simulink model "sysgenDDC"  (Simulink 7.7)
settings: Solver=VariableStepDiscrete  SolverMode=SingleTasking  StartTime=0.0  StopTime=0.003  RelTol=1e-3
PreLoadFcn:
  | sysgenDDC_PreLoadFcn
values from neighbouring files (symbols this model uses):
  Gz = [  340 ... (first row only)    [sysgenDDC_PreLoadFcn.m]
  Hz = [479 ... (first row only)    [sysgenDDC_PreLoadFcn.m]
  Ts = 1/40e006    (= 2.5e-08)    [sysgenDDC_PreLoadFcn.m]
undefined symbols (not defined in the file or in its folder): get, One, sided, xlGetSimulinkPeriod, xlipgetpartsetting
libraries: xbsIndex_r4 x132, dspsnks4 x2, xbsCopyrightNotice_r4 x1
(part 1 of 2)
settings Model: Creator=alexc  LastModifiedBy=douangp
settings DataIOCC: SignalLoggingName=sigsOut
settings OptimizationCC: BlockReduction=off  BooleanDataType=off  InitFltsAndDblsToZero=on
settings DebuggingCC: SaveWithParameterizedLinksMsg=none  SignalResolutionControl=TryResolveAllWithWarning  SolverPrmCheckMsg=none  MultiTaskDSMMsg=warning  MultiTaskCondExecSysMsg=none  StrictBusMsg=None
settings HardwareCC: TargetUnknown=on
settings RTWCC: IncludeERTFirstTime=on
settings GRTTargetCC: TargetFcnLib=ansi_tfl_tmw.mat

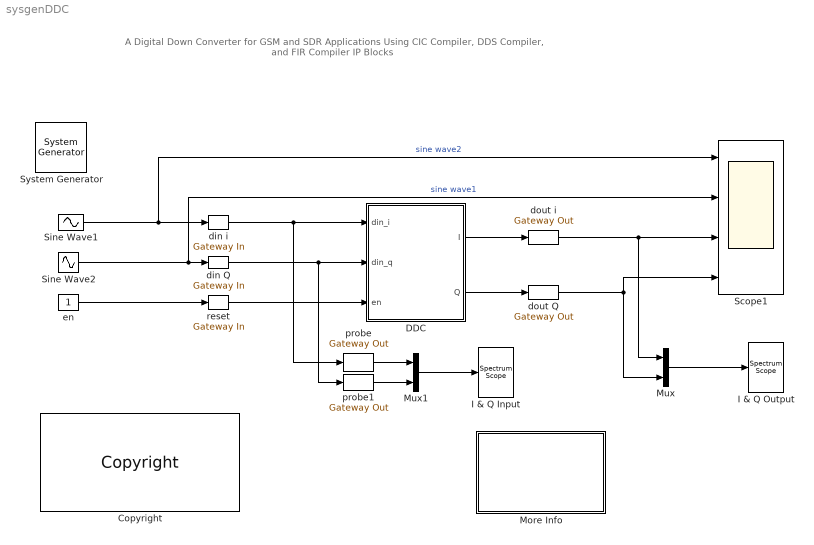
== system sysgenDDC ==
  note: A Digital Down Converter for GSM and SDR Applications
      | Using CIC Compiler, DDS Compiler, and FIR Compiler IP Blocks
  " System Generator" : xbsIndex_r4/ System Generator  Tag=genX  SystemSampleTime=-1  xilinxfamily=virtex6  part=xc6vlx240t  speed=-1  package=ff1156  synthesis_tool=XST  clock_wrapper=Clock Enables  directory=./netlist  proj_type=Project Navigator  Synth_file=XST Defaults  Impl_file=ISE Defaults  testbench=off  simulink_period=Ts  sysclk_period=6  dcm_input_clock_period=100  incr_netlist=off  trim_vbits=Everywhere in SubSystem  dbl_ovrd=According to Block Masks  core_generation=According to Block Masks  run_coregen=off  deprecated_control=off  eval_field=0  block_type=sysgen
      settings: block_version=10.1.3
  Copyright : xbsCopyrightNotice_r4/Copyright  copyrighttext="Copyright (c) 2011  by  Xilinx, Inc. All rights reserved.<br><br>This file contains proprietary, confidential information of Xilinx, Inc., is distributed under license from Xilinx, Inc., and may be used, copied and/or disclosed only pursuant to the terms of a valid license agreement with Xilinx, Inc. Xilinx hereby grants you a license to use this file solely for design, simulation, implementation and creation of design files limited to Xilinx devices or technologies. Use with non-Xilinx devices or technologies is expressly prohibited and immediately terminates your license unless covered by a separate agreement.<br><br>Xilinx is providing this design, code, or information \"as-is\" solely for use in developing programs and solutions for Xilinx devices, with no obligation on the part of Xilinx to provide support. By providing this design, code, or information as one possible implementation of this feature, application or standard, Xilinx is making no representation that this implementation is free from any claims of infringement. You are responsible for obtaining any rights you may require for your implementation. Xilinx expressly disclaims any warranty whatsoever with respect to the adequacy of the implementation, including but not limited to any warranties or representations that this implementation is free from claims of infringement, implied warranties of merchantability or fitness for a particular purpose.<br><br>Xilinx products are not intended for use in life support appliances, devices, or systems. Use in such applications is expressly prohibited.<br><br>Any modifications that are made to the Source Code are done at the user's sole risk and will be unsupported.<br><br>This copyright and support notice must be retained as part of this text at all times. (c) Copyright 1995-2011 Xilinx, Inc. All rights reserved."  block_type=copyright
      settings: block_version=9.2.00
      settings: infoedit=|
      | Copyright(C) 2007 by  Xilinx, Inc. All rights reserved.<br>
      | <br>
      | This file contains proprietary, confidential information of Xilinx, Inc., is distributed under license
      | from Xilinx, Inc., and may be used, copied and/or disclosed only pursuant to the terms of a valid license
      | agreement with Xilinx, Inc. Xilinx hereby grants you a license to use this file solely for design,
      | simulation, implementation and creation of design files limited to Xilinx devices or technologies. Use
      | with non-Xilinx devices or technologies is expressly prohibited and immediately terminates your license
      | unless covered by a separate agreement.<br>
      | <br>
      | Xilinx is providing this design, code, or information "as-is" solely for use in developing programs and
      | solutions for Xilinx devices, with no obligation on the part of Xilinx to provide support. By providing
      | this design, code, or information as one possible implementation of this feature, application or standard,
      | Xilinx is making no representation that this implementation is free from any claims of infringement. You
      | are responsible for obtaining any rights you may require for your implementation. Xilinx expressly disclaims
      | any warranty whatsoever with respect to the adequacy of the implementation, including but not limited to any
      | warranties or representations that this implementation is free from claims of infringement, implied warranties
      | of merchantability or fitness for a particular purpose.<br>
      | <br>
      | Xilinx products are not intended for use in life support appliances, devices, or systems. Use in such
      | applications is expressly prohibited.<br>
      | <br>
      | Any modifications that are made to the Source Code are done at the user's sole risk and will be unsupported.<br>
      | <br>
      | This copyright and support notice must be retained as part of this text at all times.
      | (c) Copyright 1995-2007 Xilinx, Inc. All rights reserved.
  DDC : Subsystem
  I & Q Input : dspsnks4/Spectrum Scope  SystemSampleTime=-1  ScopeProperties=off  Domain=Frequency  HorizSpan=1  UseBuffer=on  BufferSize=512  Overlap=64  TreatMby1Signals=M channels  inpFftLenInherit=off  FFTlength=128  numAvg=2  DisplayProperties=off  AxisGrid=on  Memory=off  FrameNumber=on  AxisLegend=on  AxisZoom=off  OpenScopeAtSimStart=on  OpenScopeImmediately=off  FigPos=get(0,'defaultfigureposition')  AxisProperties=on  XUnits=Hertz  XRange=One-sided ([0...Fs/2])  XDisplay=0  InheritXIncr=off  XIncr=1.0  XLabel=Samples  XLimit=Auto  YUnits=dBW/Hertz  XMax=1  XMin=0  YLabel=Magnitude, dB  LineProperties=off  LineMarkers=+  LineColors=[0 0 1]|[1 0 0]  wintypeSpecScope=Hann  RsSpecScope=50  betaSpecScope=5  winsampSpecScope=Periodic  XAxisParamsVer=6.8  isFrameUpgraded=on
      settings: YMin=-103.063615575883  YMax=27.7949833359379
  I & Q Output : dspsnks4/Spectrum Scope  SystemSampleTime=-1  ScopeProperties=off  Domain=Frequency  HorizSpan=1  UseBuffer=on  BufferSize=512  Overlap=64  TreatMby1Signals=M channels  inpFftLenInherit=off  FFTlength=128  numAvg=2  DisplayProperties=off  AxisGrid=on  Memory=off  FrameNumber=on  AxisLegend=off  AxisZoom=off  OpenScopeAtSimStart=on  OpenScopeImmediately=off  FigPos=get(0,'defaultfigureposition')  AxisProperties=on  XUnits=Hertz  XRange=One-sided ([0...Fs/2])  XDisplay=0  InheritXIncr=off  XIncr=1.0  XLabel=Samples  XLimit=Auto  YUnits=dBW/Hertz  XMax=1  XMin=0  YLabel=Magnitude, dB  LineProperties=off  LineDisables=on|on  LineStyles=--  LineMarkers=None|None  LineColors=[0 0 1]|[1 0 0]  wintypeSpecScope=Hann  RsSpecScope=50  betaSpecScope=5  winsampSpecScope=Periodic  XAxisParamsVer=6.8  isFrameUpgraded=on
      settings: YMin=-103.063615575883  YMax=27.7949833359379
  More Info : Subsystem
      mask Display: disp('Double click\n for\n more information.')
  Mux : Mux  Inputs=2
  Mux1 : Mux  Inputs=2
  Scope1 : Scope  NumInputPorts=4
      settings: TickLabels=on  YMin=-5.5e-005~-0.00025~-1~-1  YMax=0~0~1~1  SaveName=ScopeData3
  Sine Wave1 : Sin  Amplitude=1.9  Frequency=2*pi*4.975e06  SampleTime=Ts
  Sine Wave2 : Sin  Amplitude=1.9  Frequency=2*pi*5.015e06  SampleTime=Ts
  din Q : xbsIndex_r4/Gateway In  gui_display_data_type=Fixed-point  arith_type="Signed  (2's comp)"  n_bits=14  bin_pt=12  preci_type=Single  exp_width=8  frac_width=24  quantization="Round  (unbiased: +/- Inf)"  overflow=Flag as error  period=Ts  dbl_ovrd=off  timing_constraint=None  locs_specified=off  LOCs={}  hdl_port=on  block_type=gatewayin
      settings: infoedit="Gateway in block.  Converts inputs of type Simulink integer, double and fixed point to  Xilinx fixed point type.<br><br>Hardware notes:  In hardware these blocks become top level input ports."  xl_area=[0 0 0 0 14 0 0]  block_version=VER_STRING_GOES_HERE
  din i : xbsIndex_r4/Gateway In  gui_display_data_type=Fixed-point  arith_type="Signed  (2's comp)"  n_bits=14  bin_pt=12  preci_type=Single  exp_width=8  frac_width=24  quantization="Round  (unbiased: +/- Inf)"  overflow=Flag as error  period=Ts  dbl_ovrd=off  timing_constraint=None  locs_specified=off  LOCs={}  hdl_port=on  block_type=gatewayin
      settings: infoedit="Gateway in block.  Converts inputs of type Simulink integer, double and fixed point to  Xilinx fixed point type.<br><br>Hardware notes:  In hardware these blocks become top level input ports."  xl_area=[0 0 0 0 14 0 0]  block_version=VER_STRING_GOES_HERE
  dout Q : xbsIndex_r4/Gateway Out  hdl_port=on  timing_constraint="Data Rate;  Set 'FAST' Attribute"  locs_specified=off  LOCs={}  block_type=gatewayout
      settings: infoedit="Gateway out block.  Converts Xilinx fixed point inputs into ouputs of type Simulink integer, double, or fixed point.<P><P>Hardware notes:  In hardware these blocks become top level output ports or are discarded, depending on how they are configured."  xl_area=[0 0 0 0 20 0 0]  block_version=VER_STRING_GOES_HERE
  dout i : xbsIndex_r4/Gateway Out  hdl_port=on  timing_constraint="Data Rate;  Set 'FAST' Attribute"  locs_specified=off  LOCs={}  block_type=gatewayout
      settings: infoedit="Gateway out block.  Converts Xilinx fixed point inputs into ouputs of type Simulink integer, double, or fixed point.<P><P>Hardware notes:  In hardware these blocks become top level output ports or are discarded, depending on how they are configured."  xl_area=[0 0 0 0 20 0 0]  block_version=VER_STRING_GOES_HERE
  en : Constant  SampleTime=Ts
  probe : xbsIndex_r4/Gateway Out  hdl_port=off  timing_constraint="Data Rate;  Set 'FAST' Attribute"  locs_specified=off  LOCs={}  block_type=gatewayout
      settings: infoedit="Gateway out block.  Converts Xilinx fixed point inputs into ouputs of type Simulink integer, double, or fixed point.<P><P>Hardware notes:  In hardware these blocks become top level output ports or are discarded, depending on how they are configured."  xl_area=[0 0 0 0 0 0 0]  block_version=VER_STRING_GOES_HERE
  probe1 : xbsIndex_r4/Gateway Out  hdl_port=off  timing_constraint="Data Rate;  Set 'FAST' Attribute"  locs_specified=off  LOCs={}  block_type=gatewayout
      settings: infoedit="Gateway out block.  Converts Xilinx fixed point inputs into ouputs of type Simulink integer, double, or fixed point.<br><br>Hardware notes:  In hardware these blocks become top level output ports or are discarded, depending on how they are configured."  xl_area=[0 0 0 0 0 0 0]  block_version=VER_STRING_GOES_HERE
  reset : xbsIndex_r4/Gateway In  gui_display_data_type=Fixed-point  arith_type=Boolean  n_bits=24  bin_pt=0  preci_type=Single  exp_width=8  frac_width=24  quantization=Truncate  overflow=Wrap  period=Ts  dbl_ovrd=off  timing_constraint=None  locs_specified=off  LOCs={}  hdl_port=on  block_type=gatewayin
      settings: infoedit="Gateway in block.  Converts inputs of type Simulink integer, double and fixed point to  Xilinx fixed point type.<br><br>Hardware notes:  In hardware these blocks become top level input ports."  block_version=VER_STRING_GOES_HERE
  wires:
  Sine Wave1/1 -> Scope1/1, din i/1  "sine wave2"
  DDC/1(I) -> dout i/1
  DDC/2(Q) -> dout Q/1
  Sine Wave2/1 -> din Q/1, Scope1/2  "sine wave1"
  din Q/1 -> DDC/2(din_q), probe1/1
  din i/1 -> probe/1, DDC/1(din_i)
  dout i/1 -> Scope1/3, Mux/1
  dout Q/1 -> Scope1/4, Mux/2
  Mux/1 -> I & Q Output/1
  Mux1/1 -> I & Q Input/1
  probe/1 -> Mux1/1
  probe1/1 -> Mux1/2
  en/1 -> reset/1
  reset/1 -> DDC/3(en)

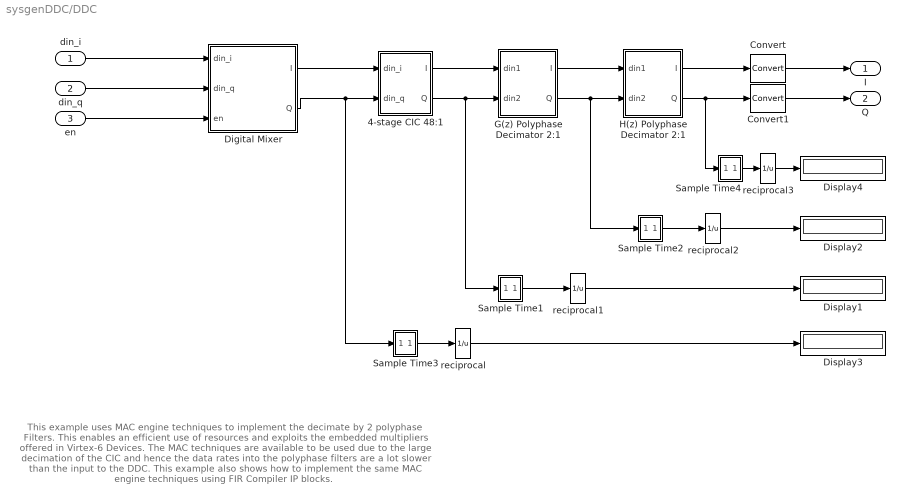
== system sysgenDDC/DDC ==
  note: This example uses MAC engine techniques to implement the decimate by 2
      | polyphase Filters. This enables an efficient use of resources and exploits the
      | embedded multipliers offered in Virtex-6 Devices. The MAC techniques are
      | available to be used due to the large decimation of the CIC and hence the data
      | rates into the polyphase filters are a lot slower than the input to the DDC.
      |
      | This example also shows how to implement the same MAC engine techniques using
      | FIR Compiler IP blocks.
  din_i : Inport
  din_q : Inport  Port=2
  en : Inport  Port=3
  4-stage CIC 48:1 : Subsystem
      mask init:
      | % Set Block Logo
      | bg = [0.3 0.8 0.3];
      | fg = [0.8 1 0.8];
      | iPos = get_param(gcb,'Position');
      | iWidth=iPos(3)-iPos(1); iHeight=iPos(4)-iPos(2);
      | iCx=iWidth/2;
      | iCy=iHeight/2;
      | [logoX, logoY] = xlogo(iPos);
      mask Display:
      | patch([0 iWidth iWidth 0],[0 0 iHeight iHeight] , bg);
      | patch(logoX,logoY , fg);
      | plot([0 0 iWidth iWidth 0], [0 iHeight iHeight 0 0]);
      | 
      | port_label('output',1,'I');
      | port_label('output',2,'Q');
  Convert : xbsIndex_r4/Convert  gui_display_data_type=Fixed-point  arith_type="Signed  (2's comp)"  n_bits=20  bin_pt=18  float_type=Single  exp_bits=8  fraction_bits=24  quantization="Round  (unbiased: +/- Inf)"  overflow=Flag as error  en=off  latency=1  dbl_ovrd=off  pipeline=off  block_type=convert
      settings: xl_area=[11 20 0 22 0 0 0]  block_version=VER_STRING_GOES_HERE
  Convert1 : xbsIndex_r4/Convert  gui_display_data_type=Fixed-point  arith_type="Signed  (2's comp)"  n_bits=20  bin_pt=18  float_type=Single  exp_bits=8  fraction_bits=24  quantization="Round  (unbiased: +/- Inf)"  overflow=Flag as error  en=off  latency=1  dbl_ovrd=off  pipeline=off  block_type=convert
      settings: xl_area=[11 20 0 22 0 0 0]  block_version=VER_STRING_GOES_HERE
  Digital Mixer : Subsystem
      mask init:
      | % Set Block Logo
      | bg = [0.3 0.8 0.3];
      | fg = [0.8 1 0.8];
      | iPos = get_param(gcb,'Position');
      | iWidth=iPos(3)-iPos(1); iHeight=iPos(4)-iPos(2);
      | iCx=iWidth/2;
      | iCy=iHeight/2;
      | [logoX, logoY] = xlogo(iPos);
      mask Display:
      | patch([0 iWidth iWidth 0],[0 0 iHeight iHeight] , bg);
      | patch(logoX,logoY , fg);
      | plot([0 0 iWidth iWidth 0], [0 iHeight iHeight 0 0]);
      | 
      | port_label('input',1,'din');
      | port_label('input',2,'din');
      | port_label('output',1,'I');
      | port_label('output',2,'Q');
  Display{1..4} (4 alike) : Display
  G(z) Polyphase Decimator 2:1 : Subsystem
      mask init:
      | % Set Block Logo
      | bg = [0.3 0.8 0.3];
      | fg = [0.8 1 0.8];
      | iPos = get_param(gcb,'Position');
      | iWidth=iPos(3)-iPos(1); iHeight=iPos(4)-iPos(2);
      | iCx=iWidth/2;
      | iCy=iHeight/2;
      | [logoX, logoY] = xlogo(iPos);
      mask Display:
      | patch([0 iWidth iWidth 0],[0 0 iHeight iHeight] , bg);
      | patch(logoX,logoY , fg);
      | plot([0 0 iWidth iWidth 0], [0 iHeight iHeight 0 0]);
      | 
      | port_label('output',1,'I');
      | port_label('output',2,'Q');
  H(z) Polyphase Decimator 2:1 : Subsystem
      mask init:
      | % Set Block Logo
      | bg = [0.3 0.8 0.3];
      | fg = [0.8 1 0.8];
      | iPos = get_param(gcb,'Position');
      | iWidth=iPos(3)-iPos(1); iHeight=iPos(4)-iPos(2);
      | iCx=iWidth/2;
      | iCy=iHeight/2;
      | [logoX, logoY] = xlogo(iPos);
      mask Display:
      | patch([0 iWidth iWidth 0],[0 0 iHeight iHeight] , bg);
      | patch(logoX,logoY , fg);
      | plot([0 0 iWidth iWidth 0], [0 iHeight iHeight 0 0]);
      | 
      | port_label('output',1,'I');
      | port_label('output',2,'Q');
  Sample Time1 : Subsystem
      settings: CopyFcn=set_param(gcb, 'LinkStatus', 'none');
      mask Display: disp('ST')
  Sample Time2 : Subsystem
      settings: CopyFcn=set_param(gcb, 'LinkStatus', 'none');
      mask Display: disp('ST')
  Sample Time3 : Subsystem
      settings: CopyFcn=set_param(gcb, 'LinkStatus', 'none');
      mask Display: disp('ST')
  Sample Time4 : Subsystem
      settings: CopyFcn=set_param(gcb, 'LinkStatus', 'none');
      mask Display: disp('ST')
  reciprocal{,1..3} (4 alike) : Math  Operator=reciprocal  SaturateOnIntegerOverflow=on
  I : Outport
  Q : Outport  Port=2
  wires:
  Digital Mixer/1(I) -> 4-stage CIC 48:1/1(din_i)
  Digital Mixer/2(Q) -> 4-stage CIC 48:1/2(din_q), Sample Time3/1(din)
  4-stage CIC 48:1/2(Q) -> Sample Time1/1(din), G(z) Polyphase Decimator 2:1/2(din2)
  Sample Time3/1(CLK) -> reciprocal/1
  Sample Time2/1(CLK) -> reciprocal2/1
  din_i/1 -> Digital Mixer/1(din_i)
  din_q/1 -> Digital Mixer/2(din_q)
  Sample Time4/1(CLK) -> reciprocal3/1
  reciprocal/1 -> Display3/1
  H(z) Polyphase Decimator 2:1/2(Q) -> Sample Time4/1(din), Convert1/1
  H(z) Polyphase Decimator 2:1/1(I) -> Convert/1
  Sample Time1/1(CLK) -> reciprocal1/1
  reciprocal1/1 -> Display1/1
  reciprocal2/1 -> Display2/1
  reciprocal3/1 -> Display4/1
  en/1 -> Digital Mixer/3(en)
  G(z) Polyphase Decimator 2:1/2(Q) -> Sample Time2/1(din), H(z) Polyphase Decimator 2:1/2(din2)
  G(z) Polyphase Decimator 2:1/1(I) -> H(z) Polyphase Decimator 2:1/1(din1)
  4-stage CIC 48:1/1(I) -> G(z) Polyphase Decimator 2:1/1(din1)
  Convert1/1 -> Q/1
  Convert/1 -> I/1

== system sysgenDDC/More Info ==
  note: Virtually all digital receivers perform channel access using a digital down-converter (DDC).
      |
      | The desired channel is translated to baseband using the digital mixer comprised
      | of multipliers, M1 and M2, and a direct digital synthesizer (DDS Compiler).  The sample rate of the
      | signal is then adjusted to match the channel bandwidth.  This is performed using a
      | multi-stage multi-rate filter consisting of  CIC Compier Filters and two polyphase decimators.  Coefficients
      | to two poyphase decimator filters are supplied by the MATLAB file (sysgenDDC_PreLoadFcn.m) and preloaded
      | when the model is open.
      |
      | The functions performed in the system are as follows:
      |   -  Waveform synthesis (DDS Compiler)
      |   - Complex multiplication
      |   - Multi-rate filtering with a combination of DDS Compiler and Polyphase decimators.
      |
      | The overall sample rate change of the DDC is 192 (48 x 2 x 2).
      | The DDS mixer signal has a spurious free dynamic range (SFDR) of 96 dB using Phase Dithering correction.
  note: A Digital Down Converter for GSM and SDR Applications

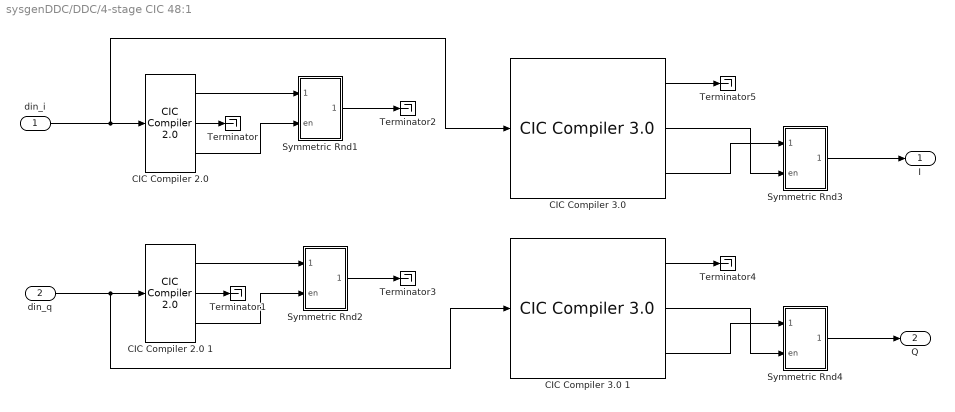
== system sysgenDDC/DDC/4-stage CIC 48:1 ==
  din_i : Inport
  din_q : Inport  Port=2
  "CIC Compiler 2.0 " : xbsIndex_r4/CIC Compiler 2.0   filter_type=Decimation  number_of_stages=4  differential_delay=1  number_of_channels=1  sample_rate_changes=Fixed  fixed_or_initial_rate=48  minimum_rate=48  maximum_rate=48  ratespecification=Maximum_Possible  sampleperiod=1  hardwareoversamplingrate=1  quantization=Full_Precision  output_data_width=41  use_xtreme_dsp_slice=on  use_streaming_interface=on  sclr=off  ce=off  gui_behaviour=Sysgen  input_data_width=18  ip_name=CIC Compiler  ip_version=2.0  dsptool_ready=true  wrapper_available=true  port_translation_map={ 'ce' => 'en', 'sclr' => 'rst' }  ipcore_xco_need_fpga_part=true  ipcore_fpga_part=xlipgetpartsetting(gcb, {'virtex4', 'xc4vsx35', '-10', 'ff668'})  ipcore_verbose=false  block_type=cic_compiler_v2_0
      settings: block_version=12.1
  CIC Compiler 2.0 1 : xbsIndex_r4/CIC Compiler 2.0   filter_type=Decimation  number_of_stages=4  differential_delay=1  number_of_channels=1  sample_rate_changes=Fixed  fixed_or_initial_rate=48  minimum_rate=4  maximum_rate=4  ratespecification=Maximum_Possible  sampleperiod=1  hardwareoversamplingrate=1  quantization=Full_Precision  output_data_width=26  use_xtreme_dsp_slice=on  use_streaming_interface=on  sclr=off  ce=off  gui_behaviour=Sysgen  input_data_width=18  ip_name=CIC Compiler  ip_version=2.0  dsptool_ready=true  wrapper_available=true  port_translation_map={ 'ce' => 'en', 'sclr' => 'rst' }  ipcore_xco_need_fpga_part=true  ipcore_fpga_part=xlipgetpartsetting(gcb, {'virtex4', 'xc4vsx35', '-10', 'ff668'})  ipcore_verbose=false  block_type=cic_compiler_v2_0
      settings: block_version=12.1
  "CIC Compiler 3.0 " : xbsIndex_r4/CIC Compiler 3.0   filter_type=Decimation  number_of_stages=4  differential_delay=1  number_of_channels=1  sample_rate_changes=Fixed  fixed_or_initial_rate=48  minimum_rate=48  maximum_rate=48  ratespecification=Maximum_Possible  sampleperiod=1  hardwareoversamplingrate=1  quantization=Full_Precision  output_data_width=41  use_xtreme_dsp_slice=on  use_streaming_interface=on  has_aclken=off  has_aresetn=off  has_dout_tready=off  trim_axipin_name=on  gui_behaviour=Sysgen_GUI  input_data_width=18  ip_name=CIC Compiler  ip_version=3.0  dsptool_ready=true  wrapper_available=true  port_translation_map={ 'aclken' => 'en', 'aresetn' => 'rst' }  ipcore_xco_need_fpga_part=true  ipcore_fpga_part=xlipgetpartsetting(gcb, {'virtex7', 'xc7v1500t', '-2', 'fhg1157'})  ipcore_verbose=false  block_type=cic_compiler_v3_0
  CIC Compiler 3.0 1 : xbsIndex_r4/CIC Compiler 3.0   filter_type=Decimation  number_of_stages=4  differential_delay=1  number_of_channels=1  sample_rate_changes=Fixed  fixed_or_initial_rate=48  minimum_rate=48  maximum_rate=48  ratespecification=Maximum_Possible  sampleperiod=1  hardwareoversamplingrate=1  quantization=Full_Precision  output_data_width=41  use_xtreme_dsp_slice=on  use_streaming_interface=on  has_aclken=off  has_aresetn=off  has_dout_tready=off  trim_axipin_name=on  gui_behaviour=Sysgen_GUI  input_data_width=18  ip_name=CIC Compiler  ip_version=3.0  dsptool_ready=true  wrapper_available=true  port_translation_map={ 'aclken' => 'en', 'aresetn' => 'rst' }  ipcore_xco_need_fpga_part=true  ipcore_fpga_part=xlipgetpartsetting(gcb, {'virtex7', 'xc7v1500t', '-2', 'fhg1157'})  ipcore_verbose=false  block_type=cic_compiler_v3_0
  Symmetric Rnd1 : Subsystem
  Symmetric Rnd2 : Subsystem
  Symmetric Rnd3 : Subsystem
  Symmetric Rnd4 : Subsystem
  Terminator{,1..5} (6 alike) : Terminator
  I : Outport
  Q : Outport  Port=2
  wires:
  CIC Compiler 2.0 1/2 -> Terminator1/1
  "CIC Compiler 2.0 "/2 -> Terminator/1
  CIC Compiler 2.0 1/3 -> Symmetric Rnd2/2(en)
  "CIC Compiler 2.0 "/3 -> Symmetric Rnd1/2(en)
  din_i/1 -> "CIC Compiler 2.0 "/1, "CIC Compiler 3.0 "/1
  CIC Compiler 2.0 1/1 -> Symmetric Rnd2/1(data)
  "CIC Compiler 2.0 "/1 -> Symmetric Rnd1/1(data)
  din_q/1 -> CIC Compiler 2.0 1/1, CIC Compiler 3.0 1/1
  Symmetric Rnd4/1(" ") -> Q/1
  Symmetric Rnd3/1(" ") -> I/1
  CIC Compiler 3.0 1/3 -> Symmetric Rnd4/1(data)
  CIC Compiler 3.0 1/2 -> Symmetric Rnd4/2(en)
  "CIC Compiler 3.0 "/3 -> Symmetric Rnd3/1(data)
  "CIC Compiler 3.0 "/2 -> Symmetric Rnd3/2(en)
  Symmetric Rnd1/1(" ") -> Terminator2/1
  Symmetric Rnd2/1(" ") -> Terminator3/1
  CIC Compiler 3.0 1/1 -> Terminator4/1
  "CIC Compiler 3.0 "/1 -> Terminator5/1

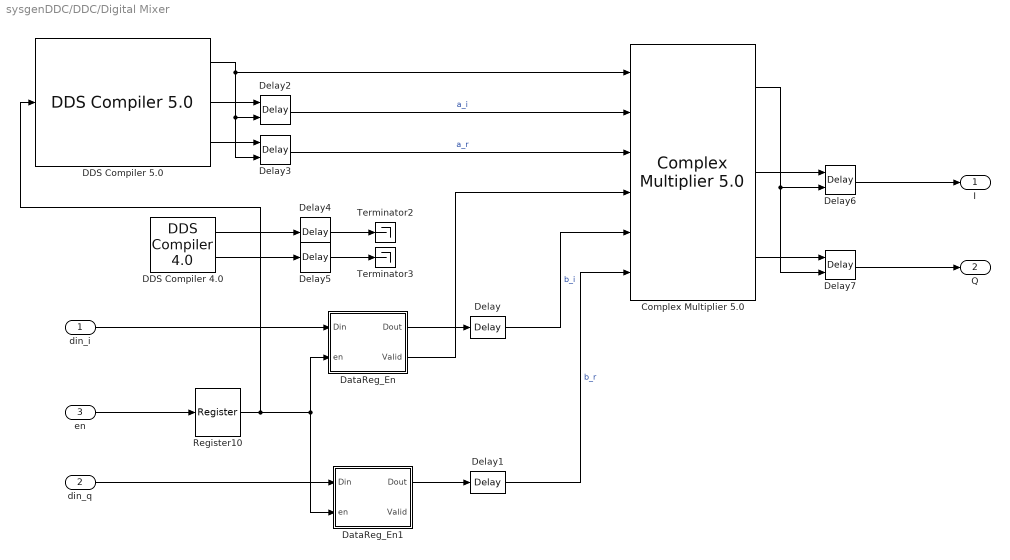
== system sysgenDDC/DDC/Digital Mixer ==
  din_i : Inport
  din_q : Inport  Port=2
  en : Inport  Port=3
  "Complex Multiplier 5.0 " : xbsIndex_r4/Complex Multiplier 5.0   hasatlast=off  hasatuser=off  atuserwidth=1  hasbtlast=off  hasbtuser=off  btuserwidth=1  multtype=Use_Mults  optimizegoal=Performance  flowcontrol=NonBlocking  outputwidth=20  roundmode=Truncate  hasctrltlast=off  hasctrltuser=off  ctrltuserwidth=1  outtlastbehv=Null  latencyconfig=Manual  minimumlatency=6  aclken=off  aresetn=off  trim_axipin_name=on  aportwidth=63  bportwidth=63  ip_name=Complex Multiplier  ip_version=5.0  dsptool_ready=true  ipcore_usecache=true  ipcore_useipmodelcache=true  ipcore_verbose=false  ipcore_latency_parameter='minimumlatency'  wrapper_available=true  port_translation_map={ 'aclken' => 'en', 'aresetn' => 'rst'}  structural_sim=false  block_type=cmpy_v5_0
  "DDS Compiler 4.0 " : xbsIndex_r4/DDS Compiler 4.0   partspresent=Phase_Generator_and_SIN_COS_LUT  dds_clock_rate=40  channels=1  parameter_entry=System_Parameters  spurious_free_dynamic_range=96  frequency_resolution=0.4  noise_shaping=Phase_Dithering  phase_width=27  output_width=16  output_selection=Sine_and_Cosine  negative_sine=off  negative_cosine=off  amplitude_mode=Full_Range  memory_type=Auto  optimization_goal=Auto  dsp48_use=Minimal  latency_configuration=Configurable  latency=1  has_phase_out=off  sclr_pin=off  clock_enable=off  rfd=off  rdy=off  channel_pin=off  explicit_period=on  period=Ts  phase_increment=Fixed  output_frequency1=4.95  output_frequency2=0  output_frequency3=0  output_frequency4=0  output_frequency5=0  output_frequency6=0  output_frequency7=0  output_frequency8=0  output_frequency9=0  output_frequency10=0  output_frequency11=0  output_frequency12=0  output_frequency13=0  output_frequency14=0  output_frequency15=0  output_frequency16=0  pinc1='111111010111000010100011'  pinc2='0'  pinc3='0'  pinc4='0'  pinc5='0'  pinc6='0'  pinc7='0'  pinc8='0'  pinc9='0'  pinc10='0'  pinc11='0'  pinc12='0'  pinc13='0'  pinc14='0'  pinc15='0'  pinc16='0'  phase_offset=None  phase_offset_angles1=0  phase_offset_angles2=0  phase_offset_angles3=0  phase_offset_angles4=0  phase_offset_angles5=0  phase_offset_angles6=0  phase_offset_angles7=0  phase_offset_angles8=0  phase_offset_angles9=0  phase_offset_angles10=0  phase_offset_angles11=0  phase_offset_angles12=0  phase_offset_angles13=0  phase_offset_angles14=0  phase_offset_angles15=0  phase_offset_angles16=0  poff1='0'  poff2='0'  poff3='0'  poff4='0'  poff5='0'  poff6='0'  poff7='0'  poff8='0'  poff9='0'  poff10='0'  poff11='0'  poff12='0'  poff13='0'  poff14='0'  poff15='0'  poff16='0'  por_mode=false  gui_behaviour=Sysgen  ip_name=DDS Compiler  ip_version=4.0  dsptool_ready=true  wrapper_available=true  port_translation_map={ 'ce' => 'en', 'sclr' => 'rst' }  ipcore_xco_need_fpga_part=true  ipcore_fpga_part=xlipgetpartsetting(gcb, {'virtex4', 'xc4vsx35', '-10', 'ff668'})  ipcore_usecache=true  ipcore_useipmodelcache=true  ipcore_verbose=false  block_type=dds_compiler_v4_0
      settings: block_version=11.3
  "DDS Compiler 5.0 " : xbsIndex_r4/DDS Compiler 5.0   partspresent=Phase_Generator_and_SIN_COS_LUT  dds_clock_rate=40  channels=1  parameter_entry=System_Parameters  spurious_free_dynamic_range=96  frequency_resolution=0.25  noise_shaping=Phase_Dithering  phase_width=27  output_width=16  output_selection=Sine_and_Cosine  negative_sine=off  negative_cosine=off  amplitude_mode=Full_Range  memory_type=Auto  optimization_goal=Auto  dsp48_use=Minimal  latency_configuration=Configurable  latency=3  has_phase_out=off  has_aclken=off  has_aresetn=off  explicit_period=on  period=Ts  data_has_tlast=Not_Required  has_tready=on  s_phase_has_tuser=Not_Required  m_data_has_tuser=Not_Required  m_phase_has_tuser=Not_Required  s_phase_tuser_width=1  s_config_sync_mode=On_Vector  phase_increment=Fixed  output_frequency1=4.95  output_frequency2=0  output_frequency3=0  output_frequency4=0  output_frequency5=0  output_frequency6=0  output_frequency7=0  output_frequency8=0  output_frequency9=0  output_frequency10=0  output_frequency11=0  output_frequency12=0  output_frequency13=0  output_frequency14=0  output_frequency15=0  output_frequency16=0  pinc1='111111010111000010100011'  pinc2='0'  pinc3='0'  pinc4='0'  pinc5='0'  pinc6='0'  pinc7='0'  pinc8='0'  pinc9='0'  pinc10='0'  pinc11='0'  pinc12='0'  pinc13='0'  pinc14='0'  pinc15='0'  pinc16='0'  phase_offset=None  phase_offset_angles1=0  phase_offset_angles2=0  phase_offset_angles3=0  phase_offset_angles4=0  phase_offset_angles5=0  phase_offset_angles6=0  phase_offset_angles7=0  phase_offset_angles8=0  phase_offset_angles9=0  phase_offset_angles10=0  phase_offset_angles11=0  phase_offset_angles12=0  phase_offset_angles13=0  phase_offset_angles14=0  phase_offset_angles15=0  phase_offset_angles16=0  poff1='0'  poff2='0'  poff3='0'  poff4='0'  poff5='0'  poff6='0'  poff7='0'  poff8='0'  poff9='0'  poff10='0'  poff11='0'  poff12='0'  poff13='0'  poff14='0'  poff15='0'  poff16='0'  trim_axipin_name=on  por_mode=false  gui_behaviour=Sysgen  ip_name=DDS Compiler  ip_version=5.0  dsptool_ready=true  wrapper_available=true  port_translation_map={ 'aclken' => 'en', 'aresetn' => 'rst' }  ipcore_xco_need_fpga_part=true  ipcore_fpga_part=xlipgetpartsetting(gcb, {'virtex6', 'xc6vlx75t', '-3', 'ff784'})  ipcore_usecache=true  ipcore_useipmodelcache=true  ipcore_verbose=false  block_type=dds_compiler_v5_0
  DataReg_En : Subsystem
  DataReg_En1 : Subsystem
  Delay : xbsIndex_r4/Delay  rst=off  infoeditControl=Selection of Reset will increase slice count due to use of real FFs and instead of SRLs  en=off  latency=0  dbl_ovrd=off  reg_retiming=off  block_type=delay
      settings: infoedit=Hardware notes: A delay line is a chain, each link of which is an SRL16 followed by a flip-flop. If register retiming is enabled, the delay line is a chain of flip-flops.  xl_area=[7 14 0 0 0 0 0]  block_version=VER_STRING_GOES_HERE
  Delay1 : xbsIndex_r4/Delay  rst=off  infoeditControl=Selection of Reset will increase slice count due to use of real FFs and instead of SRLs  en=off  latency=0  dbl_ovrd=off  reg_retiming=off  block_type=delay
      settings: infoedit=Hardware notes: A delay line is a chain, each link of which is an SRL16 followed by a flip-flop. If register retiming is enabled, the delay line is a chain of flip-flops.  xl_area=[7 14 0 0 0 0 0]  block_version=VER_STRING_GOES_HERE
  Delay{2..3,6..7} (4 alike) : xbsIndex_r4/Delay  rst=off  infoeditControl=Selection of Reset will increase slice count due to use of real FFs and instead of SRLs  en=on  latency=1  dbl_ovrd=off  reg_retiming=off  block_type=delay
  Delay4 : xbsIndex_r4/Delay  rst=off  infoeditControl=Selection of Reset will increase slice count due to use of real FFs and instead of SRLs  en=off  latency=6  dbl_ovrd=off  reg_retiming=off  block_type=delay
  Delay5 : xbsIndex_r4/Delay  rst=off  infoeditControl=Selection of Reset will increase slice count due to use of real FFs and instead of SRLs  en=off  latency=6  dbl_ovrd=off  reg_retiming=off  block_type=delay
  Register10 : xbsIndex_r4/Register  init=0  rst=off  en=off  dbl_ovrd=off  block_type=register
      settings: block_version=VER_STRING_GOES_HERE
  Terminator2 : Terminator
  Terminator3 : Terminator
  I : Outport
  Q : Outport  Port=2
  wires:
  din_i/1 -> DataReg_En/1(Din)
  DataReg_En/1(Dout) -> Delay/1
  din_q/1 -> DataReg_En1/1(Din)
  DataReg_En1/1(Dout) -> Delay1/1
  en/1 -> Register10/1
  Register10/1 -> DataReg_En/2(en), DataReg_En1/2(en), "DDS Compiler 5.0 "/1
  "DDS Compiler 5.0 "/3 -> Delay3/1
  "DDS Compiler 5.0 "/2 -> Delay2/1
  "DDS Compiler 5.0 "/1 -> Delay2/2, Delay3/2, "Complex Multiplier 5.0 "/1
  "DDS Compiler 4.0 "/1 -> Delay4/1
  "DDS Compiler 4.0 "/2 -> Delay5/1
  Delay3/1 -> "Complex Multiplier 5.0 "/3  "a_r"
  Delay6/1 -> I/1
  Delay2/1 -> "Complex Multiplier 5.0 "/2  "a_i"
  "Complex Multiplier 5.0 "/2 -> Delay6/1
  "Complex Multiplier 5.0 "/3 -> Delay7/1
  "Complex Multiplier 5.0 "/1 -> Delay7/2, Delay6/2
  Delay4/1 -> Terminator2/1
  Delay5/1 -> Terminator3/1
  Delay1/1 -> "Complex Multiplier 5.0 "/6  "b_r"
  Delay/1 -> "Complex Multiplier 5.0 "/5  "b_i"
  DataReg_En/2(Valid) -> "Complex Multiplier 5.0 "/4
  Delay7/1 -> Q/1

== system sysgenDDC/DDC/G(z) Polyphase Decimator 2:1 ==
  note: This subsystem also shows how to implement the same filter
      | using a FIR Compiler IP block
  din1 : Inport
  din2 : Inport  Port=2
  "2 Channel Decimate by 2 MAC FIR " : Subsystem  mask(2 Channel Decimate by 2 MAC FIR Filter){bit_width=18, bin_pt=16, coef1=Gz, coef2=Gz, coef_bit_width=18, coef_bin_pt=0, Ts=Ts*48}
      mask prompts: bit_width "Data Input Bit Width"; bin_pt "Data Input Binary Point"; coef1 "Coefficient Vector (Ch.1)"; coef2 "Coefficient Vector (Ch.2)"; coef_bit_width "Coefficient Bit Width"; coef_bin_pt "Coefficient Binary Point"; Ts "Sample Period"
      mask help: This is a 2 Channel Filter decimate by 2 MAC Based FIR Filter. Please setup the parameters accordingly.
      mask init:
      | %make sure there are an even number of coefficients
      | even_test1 = length(coef1)/2 - floor(length(coef1)/2);
      | if (even_test1 > 0)
      | 	coef1 = [coef1(:)' 0];
      | end
      | 
      | even_test2 = length(coef2)/2 - floor(length(coef2)/2);
      | if (even_test2 > 0)
      | 	coef2 = [coef2(:)' 0];
      | end
      | 
      | coef = 0;
      | j = 0;
      | 
      | for i = 1:2:length(coef1)
      | 
      | 	j = j+1;
      | 	coef(j) = coef1(i);
      | 
      | end
      | 
      | for i = 1:2:length(coef2)
      | 
      | 	j = j+1;
      | 	coef(j) = coef2(i);
      | 
      | end
      | 
      | for i = 2:2:length(coef1)
      | 
      | 	j = j+1;
      | 	coef(j) = coef1(i);
      | 
      | end
      | 
      | for i = 2:2:length(coef2)
      | 
      | 	j = j+1;
      | 	coef(j) = coef2(i);
      | 
      | end
      | 
      | %calculate the largest phase filter coefficient sum
      | 
      | %work in integers firstly
      | coef_int = coef*2^coef_bin_pt;
      | %Sum the coefficients
      | coef_sum1 = sum(abs(coef_int(1:length(coef_int)/4)));
      | coef_sum2 = sum(abs(coef_int(length(coef_int)/2+1:3*length(coef_int)/4)));
      | 
      | if coef_sum1 >= coef_sum2
      | 	coef_sum = coef_sum1;
      | else
      | 	coef_sum = coef_sum2;
      | end
      | 
      | %Graphic display
      | bg = [0.3 0.8 0.3];
      | fg = [0.8 1 0.8];
      | iPos = get_param(gcb,'Position');
      | iWidth=iPos(3)-iPos(1); iHeight=iPos(4)-iPos(2);
      | iCx=iWidth/2;
      | iCy=iHeight/2;
      | [logoX, logoY] = xlogo(iPos);
      mask Display:
      | patch([0 iWidth iWidth 0],[0 0 iHeight iHeight] , bg);
      | patch(logoX,logoY , fg);
      | plot([0 0 iWidth iWidth 0], [0 iHeight iHeight 0 0]);
      | 
      | disp(sprintf('2 Channel \nMAC FIR\nDecimate by 2\n%d taps',length(coef)/2) )
      | 
      | port_label ('output',1,'dout1')
      | port_label ('output',2,'dout2')
      | port_label ('input',1,'din1')
      | port_label ('input',2,'din2')
  Symmetric Round2 : Subsystem
  Symmetric Round3 : Subsystem
  I : Outport
  Q : Outport  Port=2
  wires:
  "2 Channel Decimate by 2 MAC FIR "/1(Out1) -> Symmetric Round2/1(data)
  din2/1 -> "2 Channel Decimate by 2 MAC FIR "/2(In2)
  "2 Channel Decimate by 2 MAC FIR "/2(Out2) -> Symmetric Round3/1(data)
  din1/1 -> "2 Channel Decimate by 2 MAC FIR "/1(In1)
  Symmetric Round2/1(" out") -> I/1
  Symmetric Round3/1(" out") -> Q/1

== system sysgenDDC/DDC/H(z) Polyphase Decimator 2:1 ==
  note: 96 cycles are required to implement this filter, otherwise
      | a common sample rate divisor can not be determined for
      | the design. To implement other filter sizes zeros must be
      | padded to the coefficients.
      |
      | This subsystem also shows how to implement the same filter
      | using a FIR Compiler IP block
  din1 : Inport
  din2 : Inport  Port=2
  "2 Channel Decimate by 2 MAC FIR " : Subsystem  mask(2 Channel Decimate by 2 MAC FIR Filter){bit_width=18, bin_pt=16, coef1=Hz, coef2=Hz, coef_bit_width=18, coef_bin_pt=0, Ts=Ts*96}
      mask prompts: bit_width "Data Input Bit Width"; bin_pt "Data Input Binary Point"; coef1 "Coefficient Vector (Ch.1)"; coef2 "Coefficient Vector (Ch.2)"; coef_bit_width "Coefficient Bit Width"; coef_bin_pt "Coefficient Binary Point"; Ts "Sample Period"
      mask help: This is a 2 Channel Filter decimate by 2 MAC Based FIR Filter. Please setup the parameters accordingly.
      mask init: same as sysgenDDC/DDC/G(z) Polyphase Decimator 2:1/2 Channel Decimate by 2 MAC FIR 
      mask Display:
      | patch([0 iWidth iWidth 0],[0 0 iHeight iHeight] , bg);
      | patch(logoX,logoY , fg);
      | plot([0 0 iWidth iWidth 0], [0 iHeight iHeight 0 0]);
      | 
      | disp(sprintf('2 Channel \nMAC FIR\nDecimate by 2\n%d taps',length(coef)/2) )
      | 
      | port_label ('output',1,'dout1')
      | port_label ('output',2,'dout2')
      | port_label ('input',1,'din1')
      | port_label ('input',2,'din2')
  Coarse Gain : Subsystem
  Coarse Gain1 : Subsystem
  I : Outport
  Q : Outport  Port=2
  wires:
  din1/1 -> "2 Channel Decimate by 2 MAC FIR "/1(In1)
  "2 Channel Decimate by 2 MAC FIR "/2(Out2) -> Coarse Gain1/1(data)
  din2/1 -> "2 Channel Decimate by 2 MAC FIR "/2(In2)
  "2 Channel Decimate by 2 MAC FIR "/1(Out1) -> Coarse Gain/1(data)
  Coarse Gain/1(" out") -> I/1
  Coarse Gain1/1(" out") -> Q/1

== system sysgenDDC/DDC/Sample Time1 ==
  din : Inport
  Gain : Gain  Gain=xlGetSimulinkPeriod(gcb)
  Gateway Out : xbsIndex_r4/Gateway Out  hdl_port=off  timing_constraint=None  locs_specified=off  LOCs={}  block_type=gatewayout
      settings: infoedit="Gateway out block.  Converts Xilinx fixed point inputs into ouputs of type Simulink integer, double, or fixed point.<br><br>Hardware notes:  In hardware these blocks become top level output ports or are discarded, depending on how they are configured."  block_version=11.3
  Sample Time : xbsIndex_r4/Sample Time  block_type=sampletime
      settings: infoedit=The Sample Time block reports the sample period of its input.<P><P>Hardware notes: This block is implemented as a constant in hardware.  block_version=VER_STRING_GOES_HERE
  CLK : Outport
  wires:
  Gain/1 -> CLK/1
  Sample Time/1 -> Gateway Out/1
  din/1 -> Sample Time/1
  Gateway Out/1 -> Gain/1

== system sysgenDDC/DDC/Sample Time2 ==
  din : Inport
  Gain : Gain  Gain=xlGetSimulinkPeriod(gcb)
  Gateway Out : xbsIndex_r4/Gateway Out  hdl_port=off  timing_constraint=None  locs_specified=off  LOCs={}  block_type=gatewayout
      settings: infoedit="Gateway out block.  Converts Xilinx fixed point inputs into ouputs of type Simulink integer, double, or fixed point.<br><br>Hardware notes:  In hardware these blocks become top level output ports or are discarded, depending on how they are configured."  block_version=11.3
  Sample Time : xbsIndex_r4/Sample Time  block_type=sampletime
      settings: infoedit=The Sample Time block reports the sample period of its input.<P><P>Hardware notes: This block is implemented as a constant in hardware.  block_version=VER_STRING_GOES_HERE
  CLK : Outport
  wires:
  Gain/1 -> CLK/1
  Sample Time/1 -> Gateway Out/1
  din/1 -> Sample Time/1
  Gateway Out/1 -> Gain/1

== system sysgenDDC/DDC/Sample Time3 ==
  din : Inport
  Gain : Gain  Gain=xlGetSimulinkPeriod(gcb)
  Gateway Out : xbsIndex_r4/Gateway Out  hdl_port=off  timing_constraint=None  locs_specified=off  LOCs={}  block_type=gatewayout
      settings: infoedit="Gateway out block.  Converts Xilinx fixed point inputs into ouputs of type Simulink integer, double, or fixed point.<br><br>Hardware notes:  In hardware these blocks become top level output ports or are discarded, depending on how they are configured."  block_version=11.3
  Sample Time : xbsIndex_r4/Sample Time  block_type=sampletime
      settings: infoedit=The Sample Time block reports the sample period of its input.<P><P>Hardware notes: This block is implemented as a constant in hardware.  block_version=VER_STRING_GOES_HERE
  CLK : Outport
  wires:
  Gain/1 -> CLK/1
  Sample Time/1 -> Gateway Out/1
  din/1 -> Sample Time/1
  Gateway Out/1 -> Gain/1

== system sysgenDDC/DDC/Sample Time4 ==
  din : Inport
  Gain : Gain  Gain=xlGetSimulinkPeriod(gcb)
  Gateway Out : xbsIndex_r4/Gateway Out  hdl_port=off  timing_constraint=None  locs_specified=off  LOCs={}  block_type=gatewayout
      settings: infoedit="Gateway out block.  Converts Xilinx fixed point inputs into ouputs of type Simulink integer, double, or fixed point.<br><br>Hardware notes:  In hardware these blocks become top level output ports or are discarded, depending on how they are configured."  block_version=11.3
  Sample Time : xbsIndex_r4/Sample Time  block_type=sampletime
      settings: infoedit=The Sample Time block reports the sample period of its input.<P><P>Hardware notes: This block is implemented as a constant in hardware.  block_version=VER_STRING_GOES_HERE
  CLK : Outport
  wires:
  Gain/1 -> CLK/1
  Sample Time/1 -> Gateway Out/1
  din/1 -> Sample Time/1
  Gateway Out/1 -> Gain/1

== system sysgenDDC/DDC/4-stage CIC 48:1/Symmetric Rnd1 ==
  data : Inport
  en : Inport  Port=2
  Convert : xbsIndex_r4/Convert  gui_display_data_type=Fixed-point  arith_type="Signed  (2's comp)"  n_bits=18  bin_pt=0  float_type=Single  exp_bits=8  fraction_bits=24  quantization="Round  (unbiased: +/- Inf)"  overflow=Wrap  en=off  latency=0  dbl_ovrd=off  pipeline=off  block_type=convert
      settings: xl_area=[0, 0, 0, 0, 0, 0, 0]  block_version=VER_STRING_GOES_HERE
  Register : xbsIndex_r4/Register  init=0  rst=off  en=on  dbl_ovrd=off  block_type=register
      settings: xl_area=[0, 0, 0, 0, 0, 0, 0]  block_version=VER_STRING_GOES_HERE
  Reinterpret1 : xbsIndex_r4/Reinterpret  force_arith_type=on  arith_type="Signed  (2's comp)"  force_bin_pt=on  bin_pt=24  block_type=cast
      settings: infoedit="Changes type of samples without altering their binary representation.<P><P>Hardware notes: In hardware this block costs nothing.<P><P>Example:  Suppose the input is 6 bits wide, signed, with 2 fractional bits, and the output is forced to unsigned with 0 fractional bits.  Then an input of -2.0 (1110.00 in binary 2's complement) becomes an output of 56 (111000 in binary)."  block_version=VER_STRING_GOES_HERE
  " " : Outport
  wires:
  Reinterpret1/1 -> Convert/1
  Register/1 -> " "/1
  en/1 -> Register/2
  data/1 -> Reinterpret1/1
  Convert/1 -> Register/1

== system sysgenDDC/DDC/4-stage CIC 48:1/Symmetric Rnd2 ==
  data : Inport
  en : Inport  Port=2
  Convert : xbsIndex_r4/Convert  gui_display_data_type=Fixed-point  arith_type="Signed  (2's comp)"  n_bits=18  bin_pt=0  float_type=Single  exp_bits=8  fraction_bits=24  quantization="Round  (unbiased: +/- Inf)"  overflow=Wrap  en=off  latency=0  dbl_ovrd=off  pipeline=off  block_type=convert
      settings: xl_area=[0, 0, 0, 0, 0, 0, 0]  block_version=VER_STRING_GOES_HERE
  Register : xbsIndex_r4/Register  init=0  rst=off  en=on  dbl_ovrd=off  block_type=register
      settings: xl_area=[0, 0, 0, 0, 0, 0, 0]  block_version=VER_STRING_GOES_HERE
  Reinterpret1 : xbsIndex_r4/Reinterpret  force_arith_type=on  arith_type="Signed  (2's comp)"  force_bin_pt=on  bin_pt=24  block_type=cast
      settings: infoedit="Changes type of samples without altering their binary representation.<P><P>Hardware notes: In hardware this block costs nothing.<P><P>Example:  Suppose the input is 6 bits wide, signed, with 2 fractional bits, and the output is forced to unsigned with 0 fractional bits.  Then an input of -2.0 (1110.00 in binary 2's complement) becomes an output of 56 (111000 in binary)."  block_version=VER_STRING_GOES_HERE
  " " : Outport
  wires:
  Convert/1 -> Register/1
  data/1 -> Reinterpret1/1
  en/1 -> Register/2
  Register/1 -> " "/1
  Reinterpret1/1 -> Convert/1

== system sysgenDDC/DDC/4-stage CIC 48:1/Symmetric Rnd3 ==
  data : Inport
  en : Inport  Port=2
  Convert : xbsIndex_r4/Convert  gui_display_data_type=Fixed-point  arith_type="Signed  (2's comp)"  n_bits=18  bin_pt=0  float_type=Single  exp_bits=8  fraction_bits=24  quantization="Round  (unbiased: +/- Inf)"  overflow=Wrap  en=off  latency=0  dbl_ovrd=off  pipeline=off  block_type=convert
      settings: xl_area=[0, 0, 0, 0, 0, 0, 0]  block_version=VER_STRING_GOES_HERE
  Register : xbsIndex_r4/Register  init=0  rst=off  en=on  dbl_ovrd=off  block_type=register
      settings: xl_area=[0, 0, 0, 0, 0, 0, 0]  block_version=VER_STRING_GOES_HERE
  Reinterpret1 : xbsIndex_r4/Reinterpret  force_arith_type=on  arith_type="Signed  (2's comp)"  force_bin_pt=on  bin_pt=24  block_type=cast
      settings: infoedit="Changes type of samples without altering their binary representation.<P><P>Hardware notes: In hardware this block costs nothing.<P><P>Example:  Suppose the input is 6 bits wide, signed, with 2 fractional bits, and the output is forced to unsigned with 0 fractional bits.  Then an input of -2.0 (1110.00 in binary 2's complement) becomes an output of 56 (111000 in binary)."  block_version=VER_STRING_GOES_HERE
  " " : Outport
  wires:
  Reinterpret1/1 -> Convert/1
  Register/1 -> " "/1
  en/1 -> Register/2
  data/1 -> Reinterpret1/1
  Convert/1 -> Register/1

== system sysgenDDC/DDC/4-stage CIC 48:1/Symmetric Rnd4 ==
  data : Inport
  en : Inport  Port=2
  Convert : xbsIndex_r4/Convert  gui_display_data_type=Fixed-point  arith_type="Signed  (2's comp)"  n_bits=18  bin_pt=0  float_type=Single  exp_bits=8  fraction_bits=24  quantization="Round  (unbiased: +/- Inf)"  overflow=Wrap  en=off  latency=0  dbl_ovrd=off  pipeline=off  block_type=convert
      settings: xl_area=[0, 0, 0, 0, 0, 0, 0]  block_version=VER_STRING_GOES_HERE
  Register : xbsIndex_r4/Register  init=0  rst=off  en=on  dbl_ovrd=off  block_type=register
      settings: xl_area=[0, 0, 0, 0, 0, 0, 0]  block_version=VER_STRING_GOES_HERE
  Reinterpret1 : xbsIndex_r4/Reinterpret  force_arith_type=on  arith_type="Signed  (2's comp)"  force_bin_pt=on  bin_pt=24  block_type=cast
      settings: infoedit="Changes type of samples without altering their binary representation.<P><P>Hardware notes: In hardware this block costs nothing.<P><P>Example:  Suppose the input is 6 bits wide, signed, with 2 fractional bits, and the output is forced to unsigned with 0 fractional bits.  Then an input of -2.0 (1110.00 in binary 2's complement) becomes an output of 56 (111000 in binary)."  block_version=VER_STRING_GOES_HERE
  " " : Outport
  wires:
  Convert/1 -> Register/1
  data/1 -> Reinterpret1/1
  en/1 -> Register/2
  Register/1 -> " "/1
  Reinterpret1/1 -> Convert/1

== system sysgenDDC/DDC/Digital Mixer/DataReg_En ==
  Din : Inport
  en : Inport  Port=2
  Register : xbsIndex_r4/Register  init=0  rst=off  en=on  dbl_ovrd=off  block_type=register
      settings: block_version=VER_STRING_GOES_HERE
  Register1 : xbsIndex_r4/Register  init=0  rst=off  en=off  dbl_ovrd=off  block_type=register
      settings: block_version=VER_STRING_GOES_HERE
  Dout : Outport
  Valid : Outport  Port=2
  wires:
  Din/1 -> Register/1
  Register/1 -> Dout/1
  Register1/1 -> Valid/1
  en/1 -> Register1/1, Register/2

== system sysgenDDC/DDC/Digital Mixer/DataReg_En1 ==
  Din : Inport
  en : Inport  Port=2
  Register : xbsIndex_r4/Register  init=0  rst=off  en=on  dbl_ovrd=off  block_type=register
      settings: block_version=VER_STRING_GOES_HERE
  Register1 : xbsIndex_r4/Register  init=0  rst=off  en=off  dbl_ovrd=off  block_type=register
      settings: block_version=VER_STRING_GOES_HERE
  Dout : Outport
  Valid : Outport  Port=2
  wires:
  en/1 -> Register1/1, Register/2
  Register1/1 -> Valid/1
  Register/1 -> Dout/1
  Din/1 -> Register/1
